simulink model "HardWare_bulbul"  (R2018a)
settings: Solver=VariableStepAuto  StartTime=0.0  StopTime=6  FixedStep=10e-6  RelTol=1e-3
libraries: powerlib x36, pePowerMeasurement x3, simulink x1, powerlib_meascontrol x1
settings Model: Creator=Batu  LastModifiedBy=Batu

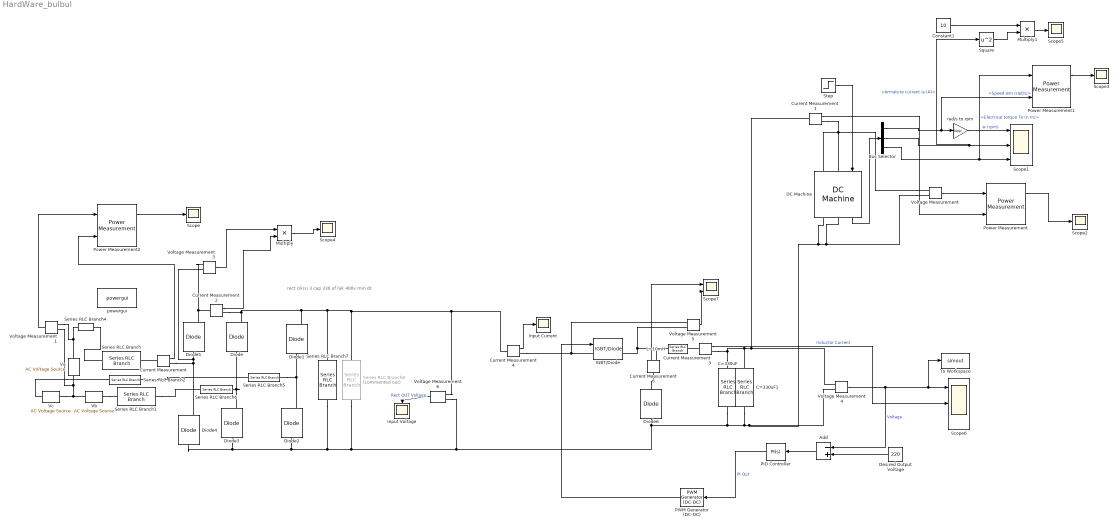
== system HardWare_bulbul ==
  note: rect cikisi 3 cap 330 uf luk 400v min dc
  " Input Current " : Scope
  Add : Sum  Inputs=-+
  Bus Selector : BusSelector  OutputSignals=Speed wm (rad/s),Armature current ia (A),Electrical torque Te (n m)
  C=330uF : powerlib/Elements/Series RLC Branch  LConnTagsString=__new0  RConnTagsString=__new0  BranchType=RC  Resistance=23e-3  Inductance=1e-3  SetiL0=off  InitialCurrent=0  Capacitance=330e-6  Setx0=off  InitialVoltage=0  Measurements=None
  C=330uF1 : powerlib/Elements/Series RLC Branch  LConnTagsString=__new0  RConnTagsString=__new0  BranchType=RC  Resistance=23e-3  Inductance=1e-3  SetiL0=off  InitialCurrent=0  Capacitance=330e-6  Setx0=off  InitialVoltage=0  Measurements=None
  Constant1 : Constant  Value=10
  Current Measurement{,1..4,6} (6 alike) : powerlib/Measurements/Current Measurement  PhasorSimulation=off  OutputType=Complex  PSBequivalent=0
  DC Machine : powerlib/Machines/DC Machine  PresetModel=No  MechanicalLoad=Torque TL  FieldType=Wound  ShowDetailedParameters=on  MeasurementBus=off  RLa="[ 10.8  12.5e-3]"  RLf="[ 210  23]"  Laf=2  MachineConstant=Back-emf constant (V/rpm)  Ke=0.3  Kt=1.8  J=1  Bm=0.01  Tf=0.01  w0=1  Ifinit=1  TsPowergui=0  TsBlock=-1
  Desired Output Voltage : Constant  Value=220
  Diode{,1..5} (6 alike) : powerlib/Power Electronics/Diode  Ron=0.02  Lon=0  Vf=0.8  IC=0  UseSnubber=0  Rs=500e6  Cs=250e-9  Measurements=on
  Diode6 : powerlib/Power Electronics/Diode  Ron=0.001  Lon=0  Vf=0.8  IC=0  UseSnubber=0  Rs=500  Cs=250e-9  Measurements=off
  IGBT/Diode : powerlib/Power Electronics/IGBT//Diode  Ron=1e-3  Rs=1e5  Cs=inf  Measurements=on
  Input Voltage : Scope
  L=10mH : powerlib/Elements/Series RLC Branch  LConnTagsString=__new0  RConnTagsString=__new0  BranchType=L  Resistance=1  Inductance=10e-3  SetiL0=off  InitialCurrent=0  Capacitance=1e-6  Setx0=off  InitialVoltage=0  Measurements=None
  Multiply : Product
  Multiply1 : Product
  PID Controller : simulink/Continuous/PID Controller  Controller=PI  TimeDomain=Continuous-time  SampleTime=-1  IntegratorMethod=Forward Euler  FilterMethod=Forward Euler  Form=Parallel  UseFilter=on  ControllerParametersSource=internal  P=4  I=10  D=0  N=100  InitialConditionSource=internal  InitialConditionForIntegrator=0  InitialConditionForFilter=0  ExternalReset=none  LimitOutput=off  UpperSaturationLimit=inf  LowerSaturationLimit=-inf  LinearizeAsGain=on  AntiWindupMode=none  Kb=1  TrackingMode=off  Kt=1  PParamMin=[]  PParamMax=[]  IParamMin=[]  IParamMax=[]  DParamMin=[]  DParamMax=[]  NParamMin=[]  NParamMax=[]  KbParamMin=[]  KbParamMax=[]  KtParamMin=[]  KtParamMax=[]  POutMin=[]  POutMax=[]  IOutMin=[]  IOutMax=[]  DOutMin=[]  DOutMax=[]  NOutMin=[]  NOutMax=[]  KbOutMin=[]  KbOutMax=[]  KtOutMin=[]  KtOutMax=[]  IntegratorOutMin=[]  IntegratorOutMax=[]  FilterOutMin=[]  FilterOutMax=[]  SumOutMin=[]  SumOutMax=[]  SumI1OutMin=[]  SumI1OutMax=[]  SumI2OutMin=[]  SumI2OutMax=[]  SumI3OutMin=[]  SumI3OutMax=[]  SumDOutMin=[]  SumDOutMax=[]  SaturationOutMin=[]  SaturationOutMax=[]  IntegratorContinuousStateAttributes=''  IntegratorStateMustResolveToSignalObject=off  IntegratorRTWStateStorageClass=Auto  FilterContinuousStateAttributes=''  FilterStateMustResolveToSignalObject=off  FilterRTWStateStorageClass=Auto  DifferentiatorICPrevScaledInput=0  DifferentiatorOutMin=[]  DifferentiatorOutMax=[]  InitialConditionSetting=State (most efficient)  FilterDiffOutCoefMin=[]  FilterDiffOutCoefMax=[]  SumDenOutMin=[]  SumDenOutMax=[]  SumNumOutMin=[]  SumNumOutMax=[]  ReciprocalOutMin=[]  ReciprocalOutMax=[]  DivideOutMin=[]  DivideOutMax=[]  TunerSelectOption=Transfer Function Based (PID Tuner App)
  PWM Generator (DC-DC) : powerlib_meascontrol/Pulse & Signal Generators/PWM Generator (DC-DC)  Fsw=500  Ts=0
  Power Measurement : pePowerMeasurement/Power Measurement  OverrideUsingVariant=Discrete  F=50  K=[0 1]  Ts=10e-6
  Power Measurement1 : pePowerMeasurement/Power Measurement  OverrideUsingVariant=Discrete  F=50  K=[0 1]  Ts=10e-6
  Power Measurement2 : pePowerMeasurement/Power Measurement  OverrideUsingVariant=Discrete  F=50  K=[0 1]  Ts=10e-6
  Scope{,2..5} (5 alike) : Scope
  Scope1 : Scope  NumInputPorts=3
  Scope6 : Scope  NumInputPorts=3
  Scope7 : Scope  NumInputPorts=2
  Series RLC Branch : powerlib/Elements/Series RLC Branch  LConnTagsString=__new0  RConnTagsString=__new0  BranchType=R  Resistance=0.1  Inductance=100e-6  SetiL0=off  InitialCurrent=0  Capacitance=1e-6  Setx0=off  InitialVoltage=0  Measurements=None
  Series RLC Branch1 : powerlib/Elements/Series RLC Branch  LConnTagsString=__new0  RConnTagsString=__new0  BranchType=R  Resistance=0.1  Inductance=100e-6  SetiL0=off  InitialCurrent=0  Capacitance=1e-6  Setx0=off  InitialVoltage=0  Measurements=None
  Series RLC Branch2 : powerlib/Elements/Series RLC Branch  LConnTagsString=__new0  RConnTagsString=__new0  BranchType=R  Resistance=0.1  Inductance=100e-6  SetiL0=off  InitialCurrent=0  Capacitance=1e-6  Setx0=off  InitialVoltage=0  Measurements=None
  Series RLC Branch4 : powerlib/Elements/Series RLC Branch  LConnTagsString=__new0  RConnTagsString=__new0  BranchType=L  Resistance=1  Inductance=100e-6  SetiL0=off  InitialCurrent=0  Capacitance=1e-6  Setx0=off  InitialVoltage=0  Measurements=None
  Series RLC Branch5 : powerlib/Elements/Series RLC Branch  LConnTagsString=__new0  RConnTagsString=__new0  BranchType=L  Resistance=1  Inductance=100e-6  SetiL0=off  InitialCurrent=0  Capacitance=1e-6  Setx0=off  InitialVoltage=0  Measurements=None
  Series RLC Branch6 : powerlib/Elements/Series RLC Branch  LConnTagsString=__new0  RConnTagsString=__new0  BranchType=L  Resistance=1  Inductance=100e-6  SetiL0=off  InitialCurrent=0  Capacitance=1e-6  Setx0=off  InitialVoltage=0  Measurements=None
  Series RLC Branch7 : powerlib/Elements/Series RLC Branch  LConnTagsString=__new0  RConnTagsString=__new0  BranchType=C  Resistance=1  Inductance=1e-3  SetiL0=off  InitialCurrent=0  Capacitance=1e-3  Setx0=off  InitialVoltage=0  Measurements=None
  Series RLC Branch8 : powerlib/Elements/Series RLC Branch  Commented=on  LConnTagsString=__new0  RConnTagsString=__new0  BranchType=C  Resistance=1  Inductance=1e-3  SetiL0=off  InitialCurrent=0  Capacitance=1e-3  Setx0=off  InitialVoltage=0  Measurements=None
  Square : Math  Operator=square  SaturateOnIntegerOverflow=on
  Step : Step  Time=0.1  After=25  SampleTime=0
  To Workspace : ToWorkspace  VariableName=simout  SampleTime=-1
  Va : powerlib/Electrical Sources/AC Voltage Source  Amplitude=240  Phase=0  Frequency=50  SampleTime=0  Measurements=None  BusType=swing  Pref=10e3  Qref=0  Qmin=-inf  Qmax=+inf
  Vb : powerlib/Electrical Sources/AC Voltage Source  Amplitude=240  Phase=240  Frequency=50  SampleTime=0  Measurements=None  BusType=swing  Pref=10e3  Qref=0  Qmin=-inf  Qmax=+inf
  Vc : powerlib/Electrical Sources/AC Voltage Source  Amplitude=240  Phase=120  Frequency=50  SampleTime=0  Measurements=None  BusType=swing  Pref=10e3  Qref=0  Qmin=-inf  Qmax=+inf
  Voltage Measurement{,1,3..6} (6 alike) : powerlib/Measurements/Voltage Measurement  PhasorSimulation=off  OutputType=Complex  PSBequivalent=0
  powergui : powerlib/powergui  Priority=1  SimulationMode=Discrete  SampleTime=10e-6  frequency=60  Iterations=50  frequencyindice=0  Pbase=100e6  ErrMax=1e-4  UnitsV=kV  UnitsW=MW  buscounter=0  FunctionMessages=off  echomessages=off  EnableUseOfTLC=off  CurrentSourceSwitches=off  DisableSnubberDevices=off  DisableRonSwitches=off  DisableVfSwitches=off  DisplayEquations=off  SolverType=Tustin/Backward Euler (TBE)  Interpol=off  ExternalGateDelay=off  methode=off  Ts=100  x0status=blocks  SPID=on  SwTol=0  HookPort=off  RestoreLinks=warning  ResistiveCurrentMeasurement=off  Frange=[0:2:500]  Ylog=off  Xlog=on  ShowGrid=off  save=off  variable=ZData  structure=0  ZoomFFT=off  StartTime=0.0  cycles=1  DisplayStyle=1  fundamental=60  FreqAxis=off  MaxFrequency=1000  frequencyindicesteady=1  RmsSteady=1  display=off
  rad/s to rpm : Gain  Gain=30/pi
  wires:
  Step/1 -> DC Machine/1
  DC Machine/1 -> Bus Selector/1
  Bus Selector/1 -> Power Measurement1/2, rad/s to rpm/1  "<Speed wm (rad/s)>"
  rad/s to rpm/1 -> Scope1/1  "w (rpm)"
  Bus Selector/2 -> Square/1, Scope1/2  "<Armature current ia (A)>"
  Bus Selector/3 -> Power Measurement1/1, Scope1/3  "<Electrical torque Te (n m)>"
  Power Measurement/1 -> Scope2/1
  Power Measurement1/1 -> Scope3/1
  Power Measurement2/1 -> Scope/1
  Current Measurement/1 -> Power Measurement2/2
  Current Measurement2/1 -> Multiply/2
  Voltage Measurement3/1 -> Multiply/1
  Multiply/1 -> Scope4/1
  Constant1/1 -> Multiply1/1
  Square/1 -> Multiply1/2
  Multiply1/1 -> Scope5/1
  Voltage Measurement1/1 -> Power Measurement2/1
  Current Measurement4/1 -> " Input Current "/1
  Current Measurement6/1 -> Scope7/1
  Voltage Measurement5/1 -> Scope7/2
  Desired Output Voltage/1 -> Add/2
  PID Controller/1 -> PWM Generator (DC-DC)/1  "PI Out"
  Voltage Measurement4/1 -> To Workspace/1, Scope6/1, Add/1  "Voltage"
  PWM Generator (DC-DC)/1 -> IGBT/Diode/1
  Voltage Measurement6/1 -> Input Voltage/1  "Rect OUT Voltage"
  Add/1 -> PID Controller/1
  Current Measurement3/1 -> Scope6/2  "Inductor Current"
  Voltage Measurement/1 -> Power Measurement/1
  Current Measurement1/1 -> Power Measurement/2
  connections:
  Vc/RConn1 -- Series RLC Branch2/LConn1
  DC Machine/RConn2 -- Voltage Measurement4/LConn2 -- C=330uF1/RConn1 -- C=330uF/RConn1 -- Voltage Measurement6/LConn2 -- Series RLC Branch8/RConn1 -- Series RLC Branch7/RConn1 -- Diode4/LConn1 -- Diode3/LConn1 -- Diode2/LConn1 -- Diode6/LConn1 -- Voltage Measurement/LConn2 -- DC Machine/RConn1
  Diode3/RConn1 -- Diode/LConn1 -- Series RLC Branch6/RConn1
  DC Machine/LConn1 -- DC Machine/LConn2 -- Current Measurement1/RConn1 -- Voltage Measurement/LConn1
  Diode4/RConn1 -- Current Measurement/RConn1 -- Voltage Measurement3/LConn1 -- Diode5/LConn1
  Vb/LConn1 -- Vc/LConn1 -- Voltage Measurement1/LConn2 -- Va/LConn1
  Va/RConn1 -- Voltage Measurement1/LConn1 -- Series RLC Branch4/LConn1
  Vb/RConn1 -- Series RLC Branch1/LConn1
  Diode2/RConn1 -- Series RLC Branch5/RConn1 -- Diode1/LConn1
  Series RLC Branch2/RConn1 -- Series RLC Branch5/LConn1
  Series RLC Branch1/RConn1 -- Series RLC Branch6/LConn1
  Series RLC Branch4/RConn1 -- Series RLC Branch/LConn1
  Current Measurement/LConn1 -- Series RLC Branch/RConn1
  Series RLC Branch7/LConn1 -- Voltage Measurement6/LConn1 -- Current Measurement4/LConn1 -- Series RLC Branch8/LConn1 -- Current Measurement2/RConn1 -- Diode/RConn1 -- Diode1/RConn1
  Diode5/RConn1 -- Voltage Measurement3/LConn2 -- Current Measurement2/LConn1
  Current Measurement4/RConn1 -- IGBT/Diode/LConn1 -- Voltage Measurement5/LConn1
  L=10mH/LConn1 -- Current Measurement6/RConn1 -- IGBT/Diode/RConn1 -- Voltage Measurement5/LConn2
  C=330uF/LConn1 -- C=330uF1/LConn1 -- Current Measurement1/LConn1 -- Voltage Measurement4/LConn1 -- Current Measurement3/RConn1
  Diode6/RConn1 -- Current Measurement6/LConn1
  Current Measurement3/LConn1 -- L=10mH/RConn1
